simulink model "simple_control"  (R2026a)
settings: Solver=VariableStepAuto  StopTime=1000
undefined symbols (not defined in the file): ekf_param, pf_param, plant_param, r_param, random_seed, u_noise_param
libraries: lib_sensors x6, lib_plant x1
settings Model: Creator=alessandro-nardin  LastModifiedBy=alessandro-nardin
settings RTWCC: Toolchain=Microsoft Visual C++ 2022 v17.0 | nmake (64-bit Windows)

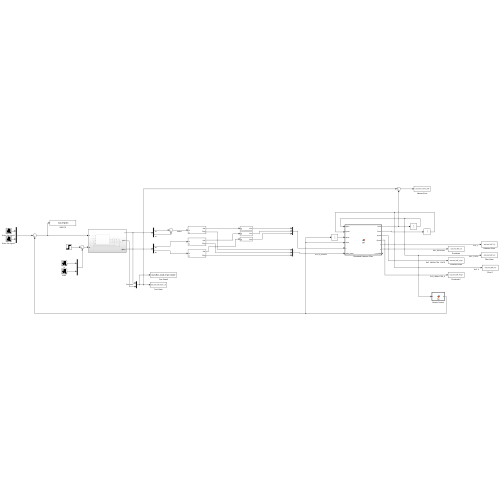
[thumbnail: Simulink's stored preview of the top-level diagram]
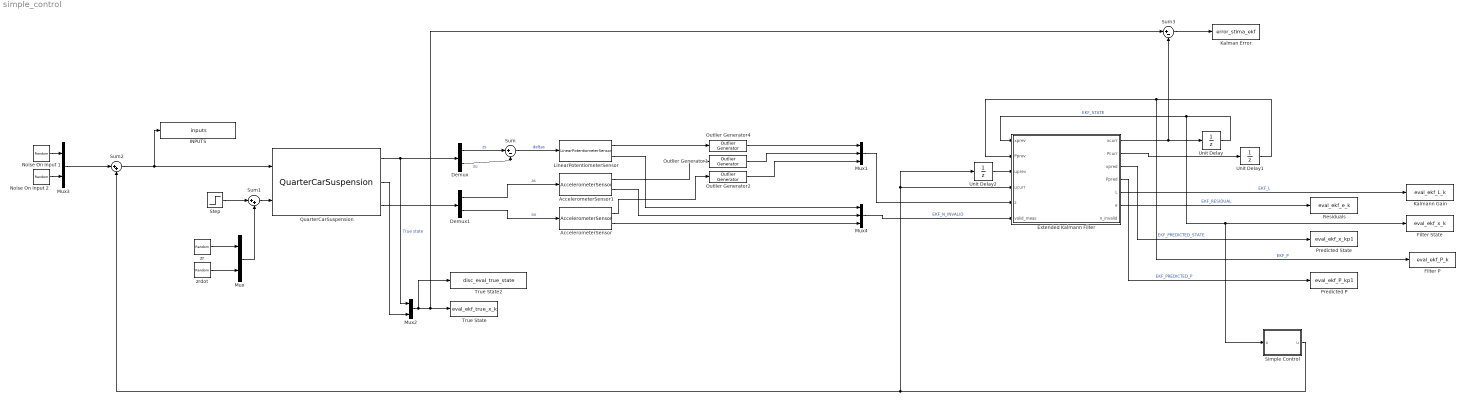
== system simple_control ==
  AccelerometerSensor : lib_sensors/AccelerometerSensor  out_sample_t=ekf_param.sample_t
  AccelerometerSensor1 : lib_sensors/AccelerometerSensor  out_sample_t=ekf_param.sample_t
  Demux : Demux  Outputs=2
  Demux1 : Demux  Outputs=2
  Extended Kalmann Filter : MATLAB Function  TreatAsAtomicUnit=on
  Filter P : ToWorkspace  VariableName=eval_ekf_P_k  SaveFormat=Timeseries  SampleTime=1/ekf_param.freq
  Filter State : ToWorkspace  VariableName=eval_ekf_x_k  SaveFormat=Timeseries  SampleTime=1/ekf_param.freq
  INPUTS : ToWorkspace  VariableName=inputs  SaveFormat=Timeseries  SampleTime=ekf_param.sample_t
  Kalman Error : ToWorkspace  VariableName=error_stima_ekf  SaveFormat=Timeseries  SampleTime=pf_param.sample_t
  Kalmann Gain : ToWorkspace  VariableName=eval_ekf_L_k  SaveFormat=Timeseries  SampleTime=pf_param.sample_t
  LinearPotentiometerSensor : lib_sensors/LinearPotentiometerSensor  out_sample_t=ekf_param.sample_t
  Mux : Mux  Inputs=2
  Mux1 : Mux  Inputs=3
  Mux2 : Mux  Inputs=2
  Mux3 : Mux  Inputs=2
  Mux4 : Mux  Inputs=3
  Noise On Input 1 : RandomNumber  Variance=u_noise_param.u1_var  Seed=random_seed+10  SampleTime=0
  Noise On Input 2 : RandomNumber  Variance=u_noise_param.u2_var  Seed=random_seed+10  SampleTime=0
  Outlier Generator1 : lib_sensors/Outlier Generator  outlier_probability=0.002  outlier_amplitude=5  sample_time=acc_param.sample_t
      settings: SourceProductName=Lib Sensors
  Outlier Generator2 : lib_sensors/Outlier Generator  outlier_probability=0.002  outlier_amplitude=5  sample_time=acc_param.sample_t
      settings: SourceProductName=Lib Sensors
  Outlier Generator4 : lib_sensors/Outlier Generator  outlier_probability=0.002  outlier_amplitude=5  sample_time=lpot_param.sample_t
      settings: SourceProductName=Lib Sensors
  Predicted P : ToWorkspace  VariableName=eval_ekf_P_kp1  SaveFormat=Timeseries  SampleTime=1/ekf_param.freq
  Predicted State : ToWorkspace  VariableName=eval_ekf_x_kp1  SaveFormat=Timeseries  SampleTime=1/ekf_param.freq
  QuarterCarSuspension : lib_plant/QuarterCarSuspension  SystemSampleTime=-1  VariantActivationTime=update diagram  EmptyChoice=off  PassThrough=off  PassThroughVariantControl=(default)  EmptyChoiceVariantControl=(default)  AllowFlexibleInterface=on  Latency=0  AutoFrameSizeCalculation=off
      settings: SourceProductName=Lib Plant
  Residuals : ToWorkspace  VariableName=eval_ekf_e_k  SaveFormat=Timeseries  SampleTime=-1
  Simple Control : MATLAB Function  TreatAsAtomicUnit=on
  Step : Step  Time=500  FinalValue=5  SampleTime=0
  Sum : Sum  Inputs=|+-
  Sum1 : Sum  Inputs=|++
  Sum2 : Sum  Inputs=|++
  Sum3 : Sum  Inputs=|+-
  True State : ToWorkspace  VariableName=eval_ekf_true_x_k  SaveFormat=Timeseries  SampleTime=1/ekf_param.freq
  True State2 : ToWorkspace  VariableName=disc_eval_true_state  SaveFormat=Timeseries  SampleTime=ekf_param.sample_t
  Unit Delay : UnitDelay  InitialCondition=ekf_param.x_init  SampleTime=ekf_param.sample_t
  Unit Delay1 : UnitDelay  InitialCondition=ekf_param.P_init  SampleTime=ekf_param.sample_t
  Unit Delay2 : UnitDelay  InitialCondition=[ 0; 0]  SampleTime=ekf_param.sample_t
  zr : RandomNumber  Variance=r_param.rz_var  Seed=random_seed+6  SampleTime=0
  zrdot : RandomNumber  Variance=r_param.rzdot_var  Seed=random_seed+7  SampleTime=0
  wires:
  Demux/1 -> Sum/1  "zs"
  Demux/2 -> Sum/2  "zu"
  Sum/1 -> LinearPotentiometerSensor/1  "deltas"
  Demux1/2 -> AccelerometerSensor/1  "au"
  QuarterCarSuspension/3 -> Demux1/1
  Demux1/1 -> AccelerometerSensor1/1  "as"
  Mux/1 -> Sum1/2
  Extended Kalmann Filter/2(Pcurr) -> Unit Delay1/1
  Unit Delay1/1 -> Extended Kalmann Filter/2(Pprev), Filter P/1  "EKF_P"
  Unit Delay2/1 -> Extended Kalmann Filter/3(uprev)
  AccelerometerSensor1/1 -> Outlier Generator1/1
  Mux1/1 -> Extended Kalmann Filter/5(z)
  zrdot/1 -> Mux/2
  Unit Delay/1 -> Extended Kalmann Filter/1(xprev), Simple Control/1(x), Filter State/1  "EKF_STATE"
  Extended Kalmann Filter/1(xcurr) -> Sum3/2, Unit Delay/1
  AccelerometerSensor/1 -> Outlier Generator2/1
  Mux4/1 -> Extended Kalmann Filter/6(valid_meas)  "EKF_N_INVALID"
  LinearPotentiometerSensor/2 -> Mux4/1
  AccelerometerSensor1/2 -> Mux4/2
  AccelerometerSensor/2 -> Mux4/3
  LinearPotentiometerSensor/1 -> Outlier Generator4/1
  QuarterCarSuspension/2 -> Mux2/2
  Extended Kalmann Filter/3(xpred) -> Predicted State/1  "EKF_PREDICTED_STATE"
  Extended Kalmann Filter/4(Ppred) -> Predicted P/1  "EKF_PREDICTED_P"
  Extended Kalmann Filter/5(L) -> Kalmann Gain/1  "EKF_L"
  Extended Kalmann Filter/6(e) -> Residuals/1  "EKF_RESIDUAL"
  QuarterCarSuspension/1 -> Mux2/1, Demux/1  "True state"
  Mux2/1 -> True State2/1, Sum3/1, True State/1
  Outlier Generator4/1 -> Mux1/1
  Outlier Generator1/1 -> Mux1/2
  Outlier Generator2/1 -> Mux1/3
  Simple Control/1(u) -> Extended Kalmann Filter/4(ucurr), Unit Delay2/1, Sum2/2
  Sum3/1 -> Kalman Error/1
  zr/1 -> Mux/1
  Noise On Input 1/1 -> Mux3/1
  Mux3/1 -> Sum2/1
  Noise On Input 2/1 -> Mux3/2
  Sum2/1 -> INPUTS/1, QuarterCarSuspension/1
  Sum1/1 -> QuarterCarSuspension/2
  Step/1 -> Sum1/1

== matlab function simple_control/Simple Control ==
  data: x input; u output
function u = fcn(x)
zs = x(1);
zu = x(2);
zsdot = x(3);
zudot = x(4);

u=[0;0];

zs_max = 15;
u1_max = 1000;


if zs<0
    u(1)= - zs/zs_max * u1_max;
end

== matlab function simple_control/Extended Kalmann Filter ==
  settings: updateMethod=DISCRETE  sampleTime=ekf_param.sample_t
  data: xprev input; Pprev input; uprev input; ucurr input; z input; xcurr output size=[ 4 1 ]; Pcurr output; xpred output; Ppred output; plant_param parameter; ekf_param parameter; L output; valid_meas input; e output; n_invalid output
function [ xcurr, Pcurr, xpred, Ppred, L, e, n_invalid ] = ekf( xprev, Pprev, uprev, ucurr, z, plant_param, ekf_param, valid_meas)
[xcurr, Pcurr, xpred, Ppred, L, e, n_invalid] = ekf_step( xprev, Pprev, uprev, ucurr, z, plant_param, ekf_param, valid_meas);
